simulink model "Scrambler"  (Simulink 7.7)
settings: Solver=ode45  StartTime=0.0  StopTime=10  RelTol=1e-3
PreLoadFcn:
  | EbNo = 16; Errors = 188; Bits = 1e8; M = 256; N = 64; Ts = 1/22050; InnerInterleaverBitTable;constellation;
undefined symbols (not defined in the file or in its folder): rsgenpoly
libraries: commutil2 x4, commblkcod2 x2, dspsnks4 x2, commcnvintrlv2 x2, commsequence2 x2, commdigbbndam3 x2, commchan3 x1, dspsrcs4 x1, commsink2 x1
settings Model: Creator=katsikas  LastModifiedBy=katsikas

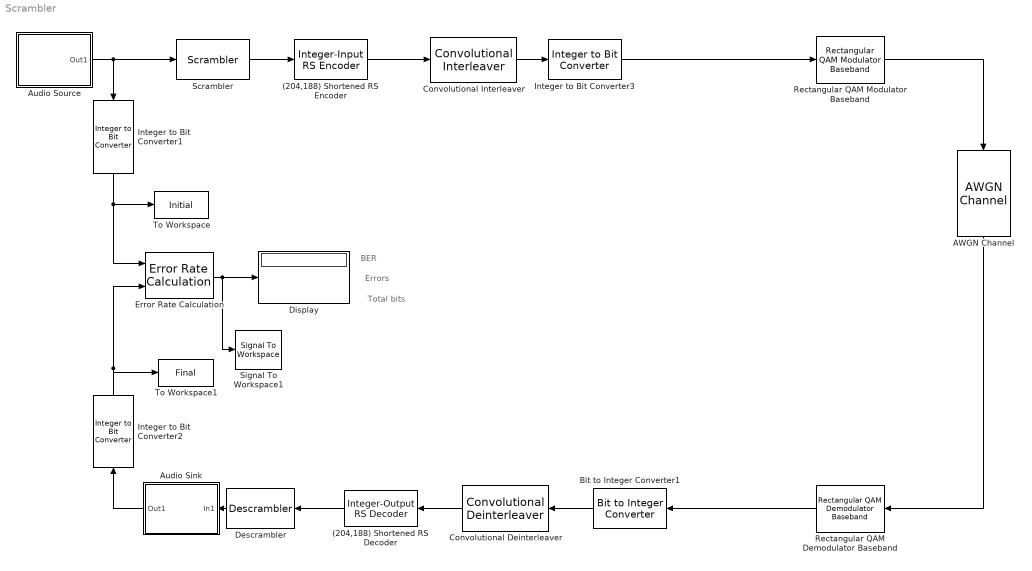
== system Scrambler ==
  note: BER
  note: Total bits
  note: Errors
  (204,188) Shortened RS Decoder : commblkcod2/Integer-Output RS Decoder  n=204  k=188  specPrimPoly=off  prPoly=[1 0 1 1]  specGenPoly=off  genPoly=rsgenpoly(7,3)  specPuncture=off  punctVec=[ones(2,1); zeros(2,1)]  specErasurePort=off  showNumErr=off
  (204,188) Shortened RS Encoder : commblkcod2/Integer-Input RS Encoder  n=204  k=188  specPrimPoly=off  prPoly=[1 0 1 1]  specGenPoly=off  genPoly=rsgenpoly(7,3)  specPuncture=off  punctVec=[ones(2,1); zeros(2,1)]
  AWGN Channel : commchan3/AWGN Channel  SystemSampleTime=-1  InputProcessing=Columns as channels (frame based)  seed=67  noiseMode="Signal to noise ratio  (Eb/No)"  EbNodB=EbNo  EsNodB=10  SNRdB=2  bitsPerSym=log2(N)  Ps=1/2048  Tsym=Ts*(188/204)  variance=1
  Audio Sink : Subsystem
  Audio Source : Subsystem
  Bit to Integer Converter1 : commutil2/Bit to Integer Converter  nbits=log2(M)  bitOrder=MSB first  signedOutputValues=Unsigned  outDtype=uint8  outDtypeSigned=Inherit via internal rule
  Convolutional Deinterleaver : commcnvintrlv2/Convolutional Deinterleaver  SystemSampleTime=-1  N=12  B=17  ic=0
  Convolutional Interleaver : commcnvintrlv2/Convolutional Interleaver  SystemSampleTime=-1  N=12  B=17  ic=0
  Descrambler : commsequence2/Descrambler  M=256  poly=[1 1 0 0 0 0 1]  ini_sta=[0]
  Display : Display
  Error Rate Calculation : commsink2/Error Rate Calculation  N=188*11*8  st_delay=0  cp_mode=Entire frame  subframe=[]  PMode=Port  WsName=ErrorVec  RsMode2=off  stop=on  numErr=Errors  maxBits=Bits
  Integer to Bit Converter1 : commutil2/Integer to Bit Converter  nbits=8  signedInputValues=Unsigned  bitOrder=MSB first  outDtype=boolean
  Integer to Bit Converter2 : commutil2/Integer to Bit Converter  nbits=8  signedInputValues=Unsigned  bitOrder=MSB first  outDtype=boolean
  Integer to Bit Converter3 : commutil2/Integer to Bit Converter  nbits=log2(M)  signedInputValues=Unsigned  bitOrder=MSB first  outDtype=boolean
  Rectangular QAM Demodulator Baseband : commdigbbndam3/Rectangular QAM Demodulator Baseband  M=N  PowType=Average Power  MinDist=2  AvgPow=1  PeakPow=1  Ph=0  Dec=User-defined  Mapping=map_constellation  OutType=Bit  DecType=Hard decision  VarSource=Dialog  Variance=1  outDtype1=boolean  outDtype2=Inherit via internal rule  derotateFactorWordLen=16  denormFactorWordLen=16  prodOutWordLen=32  prodOutRoundingMode=Floor  prodOutOverflowMode=Wrap  sumWordLen=32
  Rectangular QAM Modulator Baseband : commdigbbndam3/Rectangular QAM Modulator Baseband  M=N  InType=Bit  Enc=User-defined  Mapping=map_constellation  PowType=Average Power  MinDist=2  AvgPow=1  PeakPow=1  Ph=0  outDtype=double  outWordLen=16  outUDDataType=sfix(16)  outFracLenMode=Best precision  outFracLen=15
  Scrambler : commsequence2/Scrambler  M=256  poly=[1 1 0 0 0 0 1]  ini_sta=[0]
  Signal To Workspace1 : SignalToWorkspace  VariableName=BER  SaveFormat=Array  Save2DMode=2-D array (concatenate along first dimension)
      settings: CopyFcn=dspblkcopystw(gcbh);  MaxDataPoints=1
  To Workspace : ToWorkspace  VariableName=Initial  SampleTime=-1  SaveFormat=Array
  To Workspace1 : ToWorkspace  VariableName=Final  SampleTime=-1  SaveFormat=Array
  wires:
  Audio Source/1(Out1) -> Integer to Bit Converter1/1, Scrambler/1
  Error Rate Calculation/1 -> Display/1, Signal To Workspace1/1
  Audio Sink/1(Out1) -> Integer to Bit Converter2/1
  Integer to Bit Converter2/1 -> Error Rate Calculation/2, To Workspace1/1
  (204,188) Shortened RS Decoder/1 -> Descrambler/1
  Convolutional Deinterleaver/1 -> (204,188) Shortened RS Decoder/1
  (204,188) Shortened RS Encoder/1 -> Convolutional Interleaver/1
  Bit to Integer Converter1/1 -> Convolutional Deinterleaver/1
  Integer to Bit Converter1/1 -> Error Rate Calculation/1, To Workspace/1
  Convolutional Interleaver/1 -> Integer to Bit Converter3/1
  Rectangular QAM Modulator Baseband/1 -> AWGN Channel/1
  AWGN Channel/1 -> Rectangular QAM Demodulator Baseband/1
  Rectangular QAM Demodulator Baseband/1 -> Bit to Integer Converter1/1
  Integer to Bit Converter3/1 -> Rectangular QAM Modulator Baseband/1
  Scrambler/1 -> (204,188) Shortened RS Encoder/1
  Descrambler/1 -> Audio Sink/1(In1)

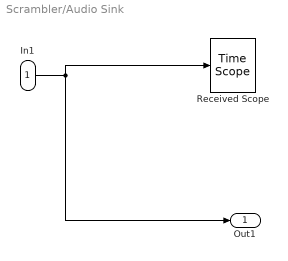
== system Scrambler/Audio Sink ==
  In1 : Inport
  Received Scope : dspsnks4/Time Scope
  Out1 : Outport
  wires:
  In1/1 -> Received Scope/1, Out1/1

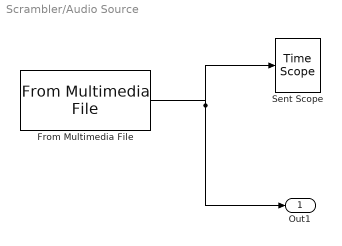
== system Scrambler/Audio Source ==
  From Multimedia File : dspsrcs4/From Multimedia File  inputFilename=speech_dft.avi  loop=on  numPlays=inf  outputStreams=Audio only  videoDataType=single  audioDataType=uint8  inheritSampleTime=on  userDefinedSampleTime=Ts  noAudioOutput=off  isIntensityVideo=off  fourcc=RGB  colorVideoFormat=Separate color signals  outputEOF=off  dataOrg=Column-major  audioFrameSize=188  computeAudioFrameSize=off
  Sent Scope : dspsnks4/Time Scope
  Out1 : Outport
  wires:
  From Multimedia File/1 -> Sent Scope/1, Out1/1
